simulink model "Rossler_habr32"  (R2014a)
settings: Solver=FixedStepDiscrete  SolverMode=SingleTasking  StartTime=0.0  StopTime=50000  RelTol=1e-3
libraries: xbsIndex_r4 x27, simulink x3
settings Model: Creator=Administrator  LastModifiedBy=Kapitanov
settings DataIOCC: SignalLoggingSaveFormat=ModelDataLogs
settings OptimizationCC: ExpressionDepthLimit=2147483647
settings DebuggingCC: UnderspecifiedInitializationDetection=Classic  FcnCallInpInsideContextMsg=UseLocalSettings  StateNameClashWarn=warning
settings GRTTargetCC: CombineOutputUpdateFcns=off  GRTInterface=on

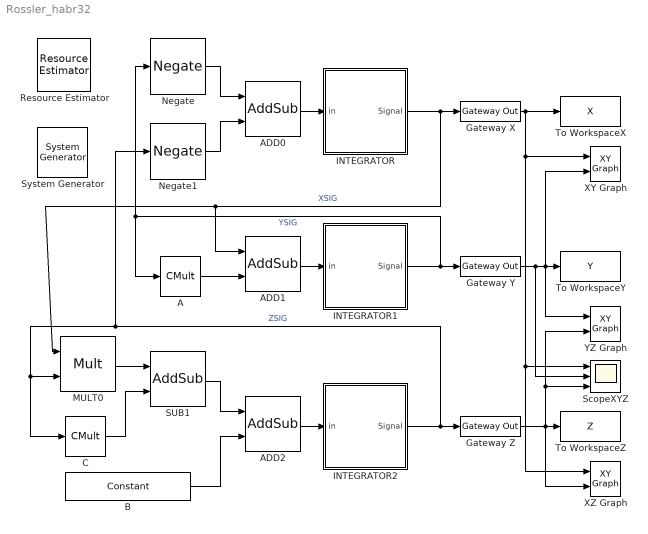
== system Rossler_habr32 ==
  " System Generator" : xbsIndex_r4/ System Generator  Tag=genX  xilinxfamily=kintex7  part=xc7k325t  speed=-3  package=fbg676  synthesis_tool=XST  clock_wrapper=Clock Enables  directory=./netlist  proj_type=Project Navigator  Synth_file=XST Defaults  Impl_file=ISE Defaults  testbench=off  simulink_period=0.01  sysclk_period=100  dcm_input_clock_period=10  incr_netlist=off  trim_vbits=Everywhere in SubSystem  dbl_ovrd=According to Block Masks  core_generation=According to Block Masks  run_coregen=off  deprecated_control=off  eval_field=0  block_type=sysgen
  A : xbsIndex_r4/CMult  const=0.2  gui_display_data_type=Fixed-point  const_n_bits=32  const_bin_pt=12  float_type=Single  exp_bits=8  fraction_bits=24  en=off  latency=0  precision=User Defined  arith_type="Signed  (2's comp)"  n_bits=64  bin_pt=52  quantization="Round  (unbiased: +/- Inf)"  overflow=Wrap  dbl_ovrd=off  use_behavioral_HDL=off  mem_type=Distributed RAM  pipeline=off  block_type=cmult
      settings: block_version=11.1
  ADD0 : xbsIndex_r4/AddSub  mode=Addition  use_carryin=off  use_carryout=off  en=off  latency=0  precision=User Defined  arith_type="Signed  (2's comp)"  n_bits=32  bin_pt=12  quantization="Round  (unbiased: +/- Inf)"  overflow=Wrap  dbl_ovrd=off  use_behavioral_HDL=off  hw_selection=Fabric  pipelined=off  block_type=addsub
      settings: block_version=11.1
  ADD1 : xbsIndex_r4/AddSub  mode=Addition  use_carryin=off  use_carryout=off  en=off  latency=0  precision=User Defined  arith_type="Signed  (2's comp)"  n_bits=32  bin_pt=12  quantization="Round  (unbiased: +/- Inf)"  overflow=Wrap  dbl_ovrd=off  use_behavioral_HDL=off  hw_selection=Fabric  pipelined=off  block_type=addsub
      settings: block_version=11.1
  ADD2 : xbsIndex_r4/AddSub  mode=Addition  use_carryin=off  use_carryout=off  en=off  latency=0  precision=User Defined  arith_type="Signed  (2's comp)"  n_bits=32  bin_pt=12  quantization="Round  (unbiased: +/- Inf)"  overflow=Wrap  dbl_ovrd=off  use_behavioral_HDL=off  hw_selection=Fabric  pipelined=off  block_type=addsub
      settings: block_version=11.1
  B : xbsIndex_r4/Constant  const=0.2  gui_display_data_type=Fixed-point  arith_type=Signed (2's comp)  n_bits=32  bin_pt=12  preci_type=Single  exp_width=8  frac_width=24  explicit_period=off  period=1  equ=P=C  opselect=C  inp2=PCIN>>17  opr=+  inp1=P  carry=CIN  dbl_ovrd=off  block_type=constant
  C : xbsIndex_r4/CMult  const=5.7  gui_display_data_type=Fixed-point  const_n_bits=32  const_bin_pt=12  float_type=Single  exp_bits=8  fraction_bits=24  en=off  latency=0  precision=User Defined  arith_type="Signed  (2's comp)"  n_bits=64  bin_pt=52  quantization="Round  (unbiased: +/- Inf)"  overflow=Wrap  dbl_ovrd=off  use_behavioral_HDL=off  mem_type=Distributed RAM  pipeline=off  block_type=cmult
      settings: block_version=11.1
  Gateway X : xbsIndex_r4/Gateway Out  inherit_from_input=off  hdl_port=on  timing_constraint=None  locs_specified=off  LOCs={}  UseAsDAC=off  DACChannel='1'  block_type=gatewayout
  Gateway Y : xbsIndex_r4/Gateway Out  inherit_from_input=off  hdl_port=on  timing_constraint=None  locs_specified=off  LOCs={}  UseAsDAC=off  DACChannel='1'  block_type=gatewayout
  Gateway Z : xbsIndex_r4/Gateway Out  inherit_from_input=off  hdl_port=on  timing_constraint=None  locs_specified=off  LOCs={}  UseAsDAC=off  DACChannel='1'  block_type=gatewayout
  INTEGRATOR : Subsystem
  INTEGRATOR1 : Subsystem
  INTEGRATOR2 : Subsystem
  MULT0 : xbsIndex_r4/Mult  precision=User Defined  arith_type="Signed  (2's comp)"  n_bits=32  bin_pt=12  quantization=Truncate  overflow=Wrap  en=off  latency=0  dbl_ovrd=off  use_behavioral_HDL=off  opt=Speed  use_embedded=on  optimum_pipeline=off  pipeline=on  use_rpm=on  placement_style=Triangular  block_type=mult
  Negate : xbsIndex_r4/Negate  precision=User Defined  arith_type="Signed  (2's comp)"  n_bits=32  bin_pt=12  quantization="Round  (unbiased: +/- Inf)"  overflow=Wrap  en=off  latency=0  dbl_ovrd=off  block_type=negate
  Negate1 : xbsIndex_r4/Negate  precision=User Defined  arith_type="Signed  (2's comp)"  n_bits=32  bin_pt=12  quantization="Round  (unbiased: +/- Inf)"  overflow=Wrap  en=off  latency=0  dbl_ovrd=off  block_type=negate
  Resource Estimator : xbsIndex_r4/Resource Estimator  Tag=resEstTag  Slices=100  FFs=500  BRAMs=20  LUTs=500  IOBs=48  EBMs=10  TBUFs=0  xl_use_estimator_area=off  est_options=Estimate  block_type=resource_estimator
      settings: AttributesFormatString=Resource\nEstimator
  SUB1 : xbsIndex_r4/AddSub  mode=Subtraction  use_carryin=off  use_carryout=off  en=off  latency=0  precision=User Defined  arith_type="Signed  (2's comp)"  n_bits=32  bin_pt=12  quantization="Round  (unbiased: +/- Inf)"  overflow=Wrap  dbl_ovrd=off  use_behavioral_HDL=off  hw_selection=Fabric  pipelined=off  block_type=addsub
      settings: block_version=11.1
  ScopeXYZ : Scope  NumInputPorts=3
      settings: Description=XYZ in time  TimeRange=5000  YMin=-20~-20~0  YMax=20~15~100  MaxDataPoints=500000
  To WorkspaceX : ToWorkspace  VariableName=X  SampleTime=0.01
  To WorkspaceY : ToWorkspace  VariableName=Y  SampleTime=0.01
  To WorkspaceZ : ToWorkspace  VariableName=Z  SampleTime=0.01
  XY Graph : simulink/Sinks/XY Graph  xmin=-30  xmax=30  ymin=-30  ymax=30  st=-1
  XZ Graph : simulink/Sinks/XY Graph  xmin=-30  xmax=30  ymin=-5  ymax=100  st=-1
  YZ Graph : simulink/Sinks/XY Graph  xmin=-30  xmax=30  ymin=-5  ymax=100  st=-1
  wires:
  INTEGRATOR/1(Signal) -> Gateway X/1, ADD1/1, MULT0/1  "XSIG"
  INTEGRATOR1/1(Signal) -> Gateway Y/1, A/1, Negate/1  "YSIG"
  ADD1/1 -> INTEGRATOR1/1(in)
  INTEGRATOR2/1(Signal) -> Gateway Z/1, MULT0/2, C/1, Negate1/1  "ZSIG"
  ADD2/1 -> INTEGRATOR2/1(in)
  Gateway X/1 -> XY Graph/1, XZ Graph/1, ScopeXYZ/1, To WorkspaceX/1
  Gateway Y/1 -> XY Graph/2, To WorkspaceY/1, YZ Graph/1, ScopeXYZ/2
  Gateway Z/1 -> To WorkspaceZ/1, XZ Graph/2, YZ Graph/2, ScopeXYZ/3
  ADD0/1 -> INTEGRATOR/1(in)
  A/1 -> ADD1/2
  MULT0/1 -> SUB1/1
  C/1 -> SUB1/2
  B/1 -> ADD2/2
  SUB1/1 -> ADD2/1
  Negate/1 -> ADD0/1
  Negate1/1 -> ADD0/2

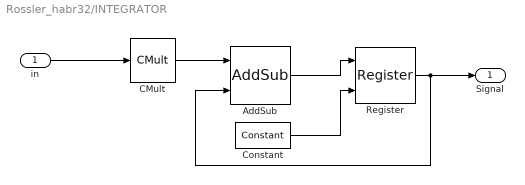
== system Rossler_habr32/INTEGRATOR ==
  in : Inport  SampleTime=0.01
  AddSub : xbsIndex_r4/AddSub  mode=Addition  use_carryin=off  use_carryout=off  en=off  latency=0  precision=User Defined  arith_type="Signed  (2's comp)"  n_bits=64  bin_pt=42  quantization="Round  (unbiased: +/- Inf)"  overflow=Wrap  dbl_ovrd=off  use_behavioral_HDL=off  hw_selection=Fabric  pipelined=off  block_type=addsub
  CMult : xbsIndex_r4/CMult  const=0.01  gui_display_data_type=Fixed-point  const_n_bits=64  const_bin_pt=42  float_type=Single  exp_bits=8  fraction_bits=24  en=off  latency=0  precision=User Defined  arith_type="Signed  (2's comp)"  n_bits=64  bin_pt=52  quantization="Round  (unbiased: +/- Inf)"  overflow=Wrap  dbl_ovrd=off  use_behavioral_HDL=off  mem_type=Distributed RAM  pipeline=off  block_type=cmult
      settings: block_version=11.1
  Constant : xbsIndex_r4/Constant  const=0  gui_display_data_type=Boolean  arith_type=Boolean  n_bits=32  bin_pt=14  preci_type=Single  exp_width=8  frac_width=24  explicit_period=on  period=1  equ=P=C  opselect=C  inp2=PCIN>>17  opr=+  inp1=P  carry=CIN  dbl_ovrd=off  block_type=constant
      settings: block_version=11.1
  Register : xbsIndex_r4/Register  init=5  rst=on  en=off  dbl_ovrd=off  block_type=register
      settings: block_version=11.1
  Signal : Outport  SampleTime=0.01
  wires:
  AddSub/1 -> Register/1
  Register/1 -> Signal/1, AddSub/2
  CMult/1 -> AddSub/1
  in/1 -> CMult/1
  Constant/1 -> Register/2

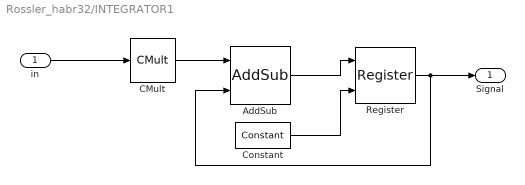
== system Rossler_habr32/INTEGRATOR1 ==
  in : Inport  SampleTime=0.01
  AddSub : xbsIndex_r4/AddSub  mode=Addition  use_carryin=off  use_carryout=off  en=off  latency=0  precision=User Defined  arith_type="Signed  (2's comp)"  n_bits=64  bin_pt=42  quantization="Round  (unbiased: +/- Inf)"  overflow=Wrap  dbl_ovrd=off  use_behavioral_HDL=off  hw_selection=Fabric  pipelined=off  block_type=addsub
  CMult : xbsIndex_r4/CMult  const=0.01  gui_display_data_type=Fixed-point  const_n_bits=64  const_bin_pt=42  float_type=Single  exp_bits=8  fraction_bits=24  en=off  latency=0  precision=User Defined  arith_type="Signed  (2's comp)"  n_bits=64  bin_pt=52  quantization="Round  (unbiased: +/- Inf)"  overflow=Wrap  dbl_ovrd=off  use_behavioral_HDL=off  mem_type=Distributed RAM  pipeline=off  block_type=cmult
      settings: block_version=11.1
  Constant : xbsIndex_r4/Constant  const=0  gui_display_data_type=Boolean  arith_type=Boolean  n_bits=32  bin_pt=14  preci_type=Single  exp_width=8  frac_width=24  explicit_period=on  period=1  equ=P=C  opselect=C  inp2=PCIN>>17  opr=+  inp1=P  carry=CIN  dbl_ovrd=off  block_type=constant
      settings: block_version=11.1
  Register : xbsIndex_r4/Register  init=-5  rst=on  en=off  dbl_ovrd=off  block_type=register
      settings: block_version=11.1
  Signal : Outport  SampleTime=0.01
  wires:
  AddSub/1 -> Register/1
  Register/1 -> Signal/1, AddSub/2
  CMult/1 -> AddSub/1
  in/1 -> CMult/1
  Constant/1 -> Register/2

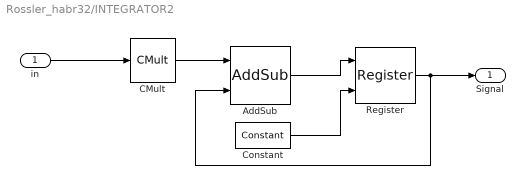
== system Rossler_habr32/INTEGRATOR2 ==
  in : Inport  SampleTime=0.01
  AddSub : xbsIndex_r4/AddSub  mode=Addition  use_carryin=off  use_carryout=off  en=off  latency=0  precision=User Defined  arith_type="Signed  (2's comp)"  n_bits=64  bin_pt=42  quantization="Round  (unbiased: +/- Inf)"  overflow=Wrap  dbl_ovrd=off  use_behavioral_HDL=off  hw_selection=Fabric  pipelined=off  block_type=addsub
  CMult : xbsIndex_r4/CMult  const=0.01  gui_display_data_type=Fixed-point  const_n_bits=64  const_bin_pt=42  float_type=Single  exp_bits=8  fraction_bits=24  en=off  latency=0  precision=User Defined  arith_type="Signed  (2's comp)"  n_bits=64  bin_pt=52  quantization="Round  (unbiased: +/- Inf)"  overflow=Wrap  dbl_ovrd=off  use_behavioral_HDL=off  mem_type=Distributed RAM  pipeline=off  block_type=cmult
      settings: block_version=11.1
  Constant : xbsIndex_r4/Constant  const=0  gui_display_data_type=Boolean  arith_type=Boolean  n_bits=32  bin_pt=14  preci_type=Single  exp_width=8  frac_width=24  explicit_period=on  period=1  equ=P=C  opselect=C  inp2=PCIN>>17  opr=+  inp1=P  carry=CIN  dbl_ovrd=off  block_type=constant
      settings: block_version=11.1
  Register : xbsIndex_r4/Register  init=0  rst=on  en=off  dbl_ovrd=off  block_type=register
      settings: block_version=11.1
  Signal : Outport  SampleTime=0.01
  wires:
  AddSub/1 -> Register/1
  Register/1 -> Signal/1, AddSub/2
  CMult/1 -> AddSub/1
  in/1 -> CMult/1
  Constant/1 -> Register/2
